simulink model "BMS"  (Simulink 8.1)
settings: Solver=ode45  StartTime=0.0  StopTime=10.0  RelTol=1e-3
libraries: simulink x1
settings Model: Creator=Brian  LastModifiedBy=Brian
settings DataIOCC: SignalLoggingSaveFormat=Dataset
settings OptimizationCC: ExpressionDepthLimit=128
settings DebuggingCC: FcnCallInpInsideContextMsg=EnableAllAsError
settings GRTTargetCC: CombineOutputUpdateFcns=on  GRTInterface=off

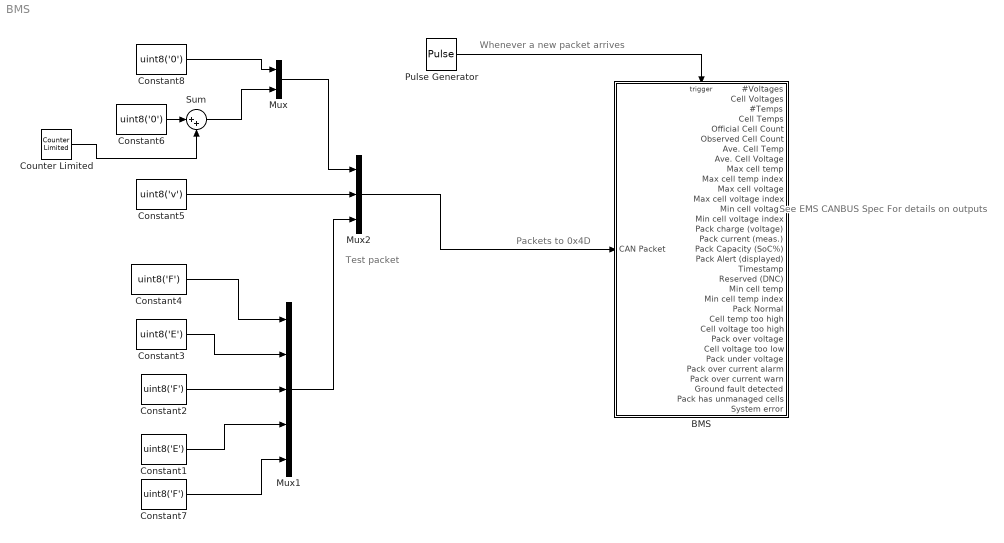
== system BMS ==
  note: Test packet
  note: See EMS
      | CANBUS Spec
      | For details on outputs
  note: Whenever a new packet arrives
  note: Packets to 0x4D
  BMS : Subsystem
  Constant1 : Constant  Value=uint8('E')  OutDataTypeStr=uint8
  Constant2 : Constant  Value=uint8('F')  OutDataTypeStr=uint8
  Constant3 : Constant  Value=uint8('E')  OutDataTypeStr=uint8
  Constant4 : Constant  Value=uint8('F')  OutDataTypeStr=uint8
  Constant5 : Constant  Value=uint8('v')  OutDataTypeStr=uint8
  Constant6 : Constant  Value=uint8('0')  OutDataTypeStr=uint8
  Constant7 : Constant  Value=uint8('F')  OutDataTypeStr=uint8
  Constant8 : Constant  Value=uint8('0')  OutDataTypeStr=uint8
  Counter Limited : simulink/Sources/Counter Limited  uplimit=9  tsamp=1
  Mux : Mux  Inputs=2
  Mux1 : Mux  Inputs=5
  Mux2 : Mux  Inputs=3
  Pulse Generator : DiscretePulseGenerator  PulseType=Time based  Period=.5  PulseWidth=5
  Sum : Sum  Inputs=|++
  wires:
  Pulse Generator/1 -> BMS/Trigger
  Constant2/1 -> Mux1/3
  Constant3/1 -> Mux1/2
  Constant4/1 -> Mux1/1
  Constant1/1 -> Mux1/4
  Constant7/1 -> Mux1/5
  Constant8/1 -> Mux/1
  Mux/1 -> Mux2/1
  Constant5/1 -> Mux2/2
  Mux1/1 -> Mux2/3
  Mux2/1 -> BMS/1(CAN Packet)
  Sum/1 -> Mux/2
  Constant6/1 -> Sum/1
  Counter Limited/1 -> Sum/2

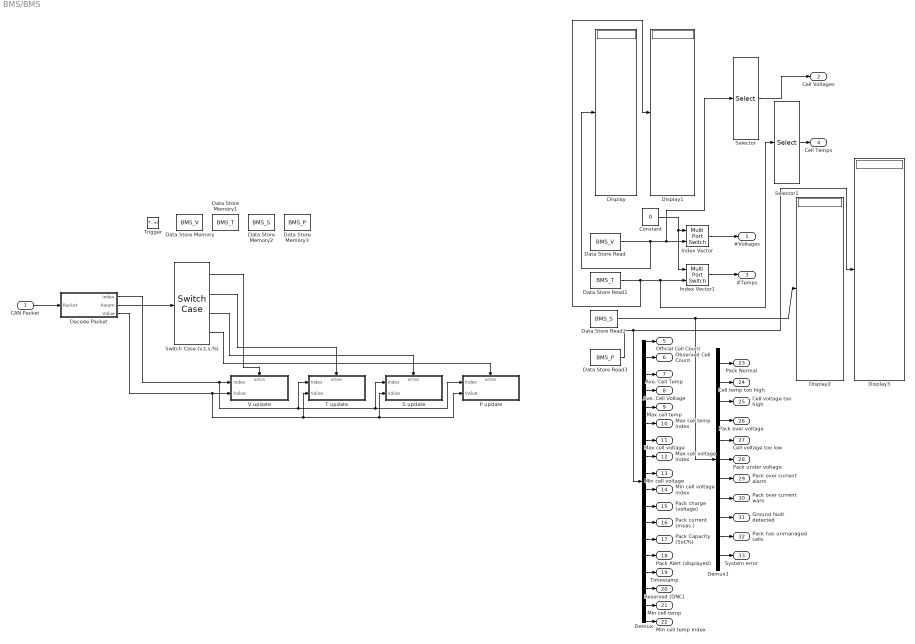
== system BMS/BMS ==
  CAN Packet : Inport
  Trigger : TriggerPort  PortDimensions=1
  Constant : Constant  Value=0
  Data Store Memory : DataStoreMemory  DataStoreName=BMS_V  ReadBeforeWriteMsg=warning  WriteAfterWriteMsg=warning  WriteAfterReadMsg=warning  InitialValue=zeros(1,hex2dec('10'))  OutDataTypeStr=uint32  Dimensions=hex2dec('10')
  Data Store Memory1 : DataStoreMemory  DataStoreName=BMS_T  ReadBeforeWriteMsg=warning  WriteAfterWriteMsg=warning  WriteAfterReadMsg=warning  InitialValue=zeros(1,hex2dec('10'))  OutDataTypeStr=uint32  Dimensions=hex2dec('10')
  Data Store Memory2 : DataStoreMemory  DataStoreName=BMS_S  ReadBeforeWriteMsg=warning  WriteAfterWriteMsg=warning  WriteAfterReadMsg=warning  InitialValue=zeros(1,11)  OutDataTypeStr=uint32  Dimensions=11
  Data Store Memory3 : DataStoreMemory  DataStoreName=BMS_P  ReadBeforeWriteMsg=warning  WriteAfterWriteMsg=warning  WriteAfterReadMsg=warning  InitialValue=zeros(1,18)  OutDataTypeStr=uint32  Dimensions=18
  Data Store Read : DataStoreRead  DataStoreName=BMS_V  DataStoreElements=BMS_V
  Data Store Read1 : DataStoreRead  DataStoreName=BMS_T  DataStoreElements=BMS_T
  Data Store Read2 : DataStoreRead  DataStoreName=BMS_S  DataStoreElements=BMS_S
  Data Store Read3 : DataStoreRead  DataStoreName=BMS_P  DataStoreElements=BMS_P
  Decode Packet : Subsystem
  Demux : Demux  Outputs=18
  Demux1 : Demux  Outputs=11
  Display{,1..3} (4 alike) : Display
      settings: Format=hex (Stored Integer)
  Index Vector : MultiPortSwitch  DataPortOrder=Zero-based contiguous  Inputs=1  zeroidx=on
  Index Vector1 : MultiPortSwitch  DataPortOrder=Zero-based contiguous  Inputs=1  zeroidx=on
  P update : Subsystem  TreatAsAtomicUnit=on
  S update : Subsystem  TreatAsAtomicUnit=on
  Selector : Selector  InputPortWidth=16  IndexOptions=Starting index (dialog)  Indices=[2]  OutputSizes=15
  Selector1 : Selector  InputPortWidth=16  IndexOptions=Starting index (dialog)  Indices=[2]  OutputSizes=15
  Switch Case (v,t,s,%) : SwitchCase  CaseConditions={uint8('v'),uint8('t'),uint8('s'),uint8('%')}  ShowDefaultCase=off
  T update : Subsystem  TreatAsAtomicUnit=on
  V update : Subsystem  TreatAsAtomicUnit=on
  #Voltages : Outport
  Cell Voltages : Outport  Port=2
  #Temps : Outport  Port=3
  Cell Temps : Outport  Port=4
  Official Cell Count : Outport  Port=5
  Observed Cell Count : Outport  Port=6
  Ave. Cell Temp : Outport  Port=7
  Ave. Cell Voltage : Outport  Port=8
  Max cell temp : Outport  Port=9
  Max cell temp index : Outport  Port=10
  Max cell voltage : Outport  Port=11
  Max cell voltage index : Outport  Port=12
  Min cell voltage : Outport  Port=13
  Min cell voltage index : Outport  Port=14
  Pack charge (voltage) : Outport  Port=15
  Pack current (meas.) : Outport  Port=16
  Pack Capacity (SoC%) : Outport  Port=17
  Pack Alert (displayed) : Outport  Port=18
  Timestamp : Outport  Port=19
  Reserved (DNC) : Outport  Port=20
  Min cell temp : Outport  Port=21
  Min cell temp index : Outport  Port=22
  Pack Normal : Outport  Port=23
  Cell temp too high : Outport  Port=24
  Cell voltage too high : Outport  Port=25
  Pack over voltage : Outport  Port=26
  Cell voltage too low : Outport  Port=27
  Pack under voltage : Outport  Port=28
  Pack over current alarm : Outport  Port=29
  Pack over current warn : Outport  Port=30
  Ground fault detected : Outport  Port=31
  "Pack has unmanaged cells " : Outport  Port=32
  System error : Outport  Port=33
  wires:
  CAN Packet/1 -> Decode Packet/1(Packet)
  Decode Packet/1(Index) -> T update/1(Index), S update/1(Index), P update/1(Index), V update/1(Index)
  Decode Packet/3(Value) -> P update/2(Value), S update/2(Value), T update/2(Value), V update/2(Value)
  Switch Case (v,t,s,%)/1 -> V update/Action
  Switch Case (v,t,s,%)/2 -> T update/Action
  Switch Case (v,t,s,%)/3 -> S update/Action
  Switch Case (v,t,s,%)/4 -> P update/Action
  Decode Packet/2(Param) -> Switch Case (v,t,s,%)/1
  Data Store Read/1 -> Display/1, Selector/1, Index Vector/2
  Data Store Read1/1 -> Selector1/1, Index Vector1/2, Display1/1
  Data Store Read2/1 -> Demux1/1, Display2/1
  Data Store Read3/1 -> Demux/1, Display3/1
  Constant/1 -> Index Vector1/1, Index Vector/1
  Index Vector/1 -> #Voltages/1
  Index Vector1/1 -> #Temps/1
  Demux/1 -> Official Cell Count/1
  Demux/2 -> Observed Cell Count/1
  Demux/3 -> Ave. Cell Temp/1
  Demux/4 -> Ave. Cell Voltage/1
  Demux/5 -> Max cell temp/1
  Demux/6 -> Max cell temp index/1
  Demux/7 -> Max cell voltage/1
  Demux/8 -> Max cell voltage index/1
  Demux/9 -> Min cell voltage/1
  Demux/10 -> Min cell voltage index/1
  Demux/11 -> Pack charge (voltage)/1
  Demux/12 -> Pack current (meas.)/1
  Demux/13 -> Pack Capacity (SoC%)/1
  Demux/14 -> Pack Alert (displayed)/1
  Demux/15 -> Timestamp/1
  Demux/16 -> Reserved (DNC)/1
  Demux/17 -> Min cell temp/1
  Demux/18 -> Min cell temp index/1
  Demux1/1 -> Pack Normal/1
  Demux1/2 -> Cell temp too high/1
  Demux1/3 -> Cell voltage too high/1
  Demux1/4 -> Pack over voltage/1
  Demux1/5 -> Cell voltage too low/1
  Demux1/6 -> Pack under voltage/1
  Demux1/7 -> Pack over current alarm/1
  Demux1/8 -> Pack over current warn/1
  Demux1/9 -> Ground fault detected/1
  Demux1/10 -> "Pack has unmanaged cells "/1
  Demux1/11 -> System error/1
  Selector/1 -> Cell Voltages/1
  Selector1/1 -> Cell Temps/1

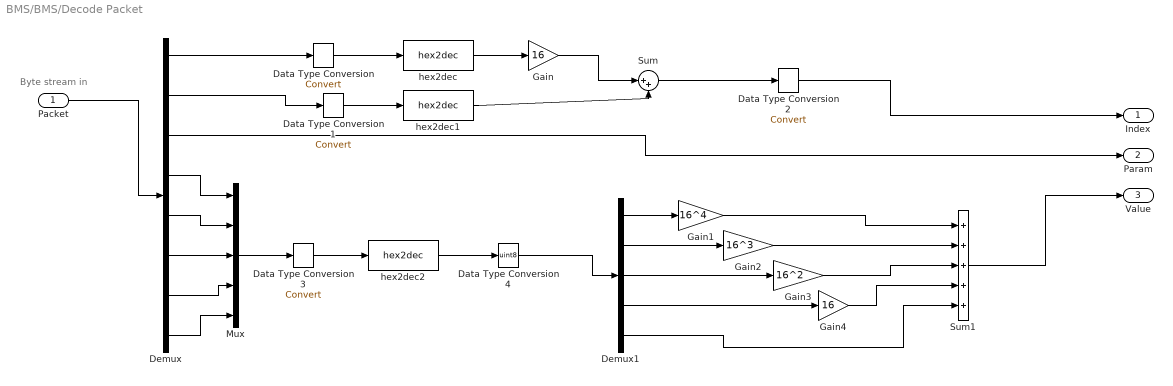
== system BMS/BMS/Decode Packet ==
  note: Byte stream in
  Packet : Inport  OutDataTypeStr=uint8
  Data Type Conversion{,1..3} (4 alike) : DataTypeConversion
  Data Type Conversion4 : DataTypeConversion  OutDataTypeStr=uint8
  Demux : Demux  Outputs=8
  Demux1 : Demux  Outputs=5
  Gain : Gain  Gain=16
  Gain1 : Gain  Gain=16^4  OutDataTypeStr=uint32
  Gain2 : Gain  Gain=16^3  OutDataTypeStr=uint32
  Gain3 : Gain  Gain=16^2  OutDataTypeStr=uint32
  Gain4 : Gain  Gain=16  OutDataTypeStr=uint32
  Mux : Mux  Inputs=5
  Sum : Sum  Inputs=|++
  Sum1 : Sum  Inputs=+++++
  hex2dec : MATLABFcn  MATLABFcn=hex2dec  OutputDimensions=1
  hex2dec1 : MATLABFcn  MATLABFcn=hex2dec  OutputDimensions=1
  hex2dec2 : MATLABFcn  MATLABFcn=hex2dec
  Index : Outport  OutDataTypeStr=uint8
  Param : Outport  Port=2  OutDataTypeStr=uint8
  Value : Outport  Port=3  OutDataTypeStr=uint32
  wires:
  Packet/1 -> Demux/1
  Demux/3 -> Param/1
  Demux/6 -> Mux/3
  Demux/7 -> Mux/4
  Demux/8 -> Mux/5
  Demux/5 -> Mux/2
  Demux/4 -> Mux/1
  Mux/1 -> Data Type Conversion3/1
  hex2dec/1 -> Gain/1
  hex2dec1/1 -> Sum/2
  Gain/1 -> Sum/1
  Sum/1 -> Data Type Conversion2/1
  Demux/1 -> Data Type Conversion/1
  Demux/2 -> Data Type Conversion1/1
  Data Type Conversion/1 -> hex2dec/1
  Data Type Conversion1/1 -> hex2dec1/1
  Data Type Conversion2/1 -> Index/1
  hex2dec2/1 -> Data Type Conversion4/1
  Data Type Conversion3/1 -> hex2dec2/1
  Data Type Conversion4/1 -> Demux1/1
  Demux1/1 -> Gain1/1
  Demux1/2 -> Gain2/1
  Demux1/3 -> Gain3/1
  Demux1/4 -> Gain4/1
  Demux1/5 -> Sum1/5
  Gain4/1 -> Sum1/4
  Gain3/1 -> Sum1/3
  Gain2/1 -> Sum1/2
  Gain1/1 -> Sum1/1
  Sum1/1 -> Value/1

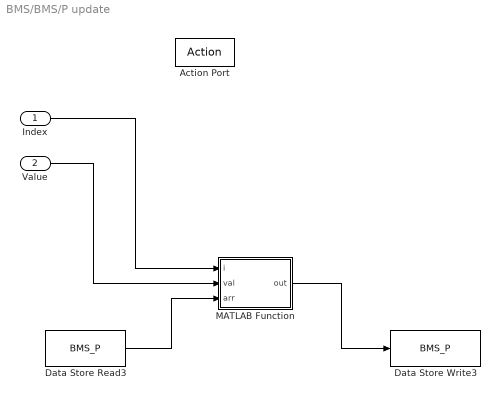
== system BMS/BMS/P update ==
  Index : Inport
  Value : Inport  Port=2
  Action Port : ActionPort  ActionType=case
  Data Store Read3 : DataStoreRead  DataStoreName=BMS_P  DataStoreElements=BMS_P
  Data Store Write3 : DataStoreWrite  DataStoreName=BMS_P  DataStoreElements=BMS_P
  MATLAB Function : MATLAB Function  TreatAsAtomicUnit=on
  wires:
  Index/1 -> MATLAB Function/1(i)
  Value/1 -> MATLAB Function/2(val)
  Data Store Read3/1 -> MATLAB Function/3(arr)
  MATLAB Function/1(out) -> Data Store Write3/1

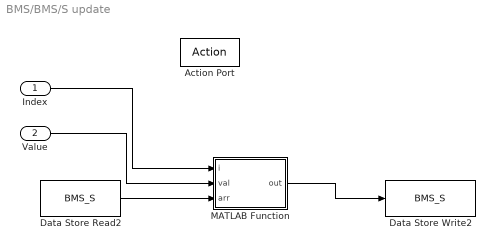
== system BMS/BMS/S update ==
  Index : Inport
  Value : Inport  Port=2
  Action Port : ActionPort  ActionType=case
  Data Store Read2 : DataStoreRead  DataStoreName=BMS_S  DataStoreElements=BMS_S
  Data Store Write2 : DataStoreWrite  DataStoreName=BMS_S  DataStoreElements=BMS_S
  MATLAB Function : MATLAB Function  TreatAsAtomicUnit=on
  wires:
  Index/1 -> MATLAB Function/1(i)
  Value/1 -> MATLAB Function/2(val)
  Data Store Read2/1 -> MATLAB Function/3(arr)
  MATLAB Function/1(out) -> Data Store Write2/1

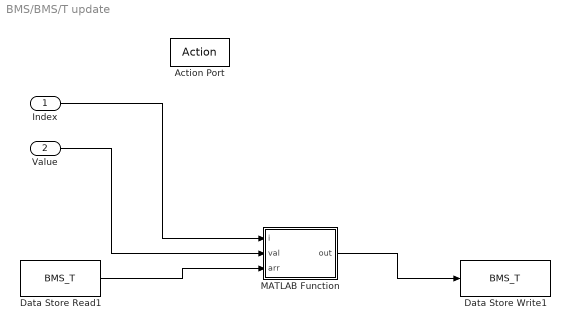
== system BMS/BMS/T update ==
  Index : Inport
  Value : Inport  Port=2
  Action Port : ActionPort  ActionType=case
  Data Store Read1 : DataStoreRead  DataStoreName=BMS_T  DataStoreElements=BMS_T
  Data Store Write1 : DataStoreWrite  DataStoreName=BMS_T  DataStoreElements=BMS_T
  MATLAB Function : MATLAB Function  TreatAsAtomicUnit=on
  wires:
  MATLAB Function/1(out) -> Data Store Write1/1
  Index/1 -> MATLAB Function/1(i)
  Value/1 -> MATLAB Function/2(val)
  Data Store Read1/1 -> MATLAB Function/3(arr)

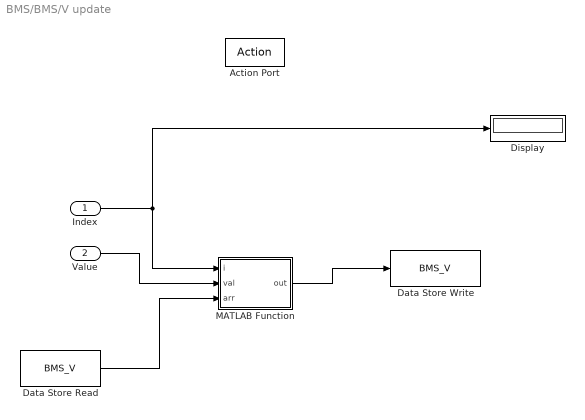
== system BMS/BMS/V update ==
  Index : Inport  OutDataTypeStr=uint8
  Value : Inport  Port=2  OutDataTypeStr=uint32
  Action Port : ActionPort  ActionType=case
  Data Store Read : DataStoreRead  DataStoreName=BMS_V  DataStoreElements=BMS_V
  Data Store Write : DataStoreWrite  DataStoreName=BMS_V  DataStoreElements=BMS_V
  Display : Display
  MATLAB Function : MATLAB Function  TreatAsAtomicUnit=on
  wires:
  Index/1 -> MATLAB Function/1(i), Display/1
  Value/1 -> MATLAB Function/2(val)
  Data Store Read/1 -> MATLAB Function/3(arr)
  MATLAB Function/1(out) -> Data Store Write/1

== matlab function BMS/T update/MATLAB Function ==
  data: i input double; out output double; val input double; arr input double
function out = fcn(i,val,arr)
%#codegen

out = arr;
out(i+1) = val;

== matlab function BMS/V update/MATLAB Function ==
  data: i input double; out output double; val input double; arr input double
function out = fcn(i,val,arr)
%#codegen

out = arr;
out(i+1) = val;

== matlab function BMS/S update/MATLAB Function ==
  data: i input double; out output double; val input double; arr input double
function out = fcn(i,val,arr)
%#codegen

out = arr;
out(i+1) = val;

== matlab function BMS/P update/MATLAB Function ==
  data: i input double; out output double; val input double; arr input double
function out = fcn(i,val,arr)
%#codegen

out = arr;
out(i+1) = val;
